simulink model "TransferFunctionAnaylsis"  (R2024a)
settings: Solver=VariableStepAuto  StartTime=0.0  StopTime=10.0  RelTol=1e-3
values from neighbouring files (symbols this model uses):
  Flux = 0.1827    [Parameters.m]    (also in StateSpace.m = 0.192)
  L_d = 0.00525    [Parameters.m]
  L_q = 0.00525    [Parameters.m]
  R_s = 0.9585    [Parameters.m]
libraries: simulink x1
settings Model: Creator=nicco  LastModifiedBy=nicco

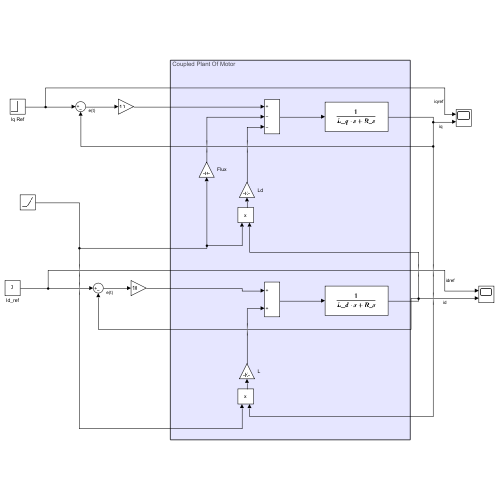
[thumbnail: Simulink's stored preview of the top-level diagram]
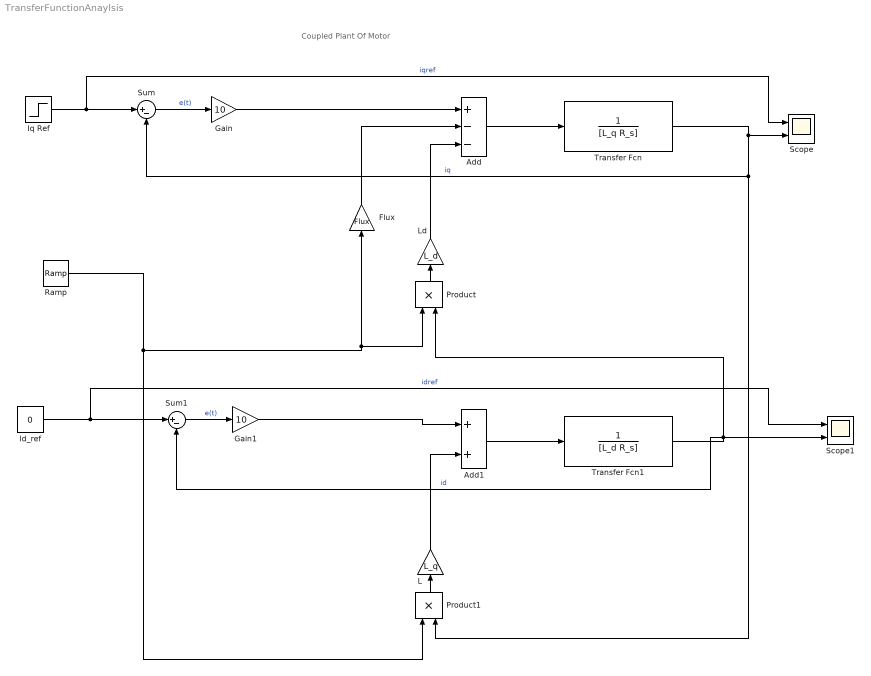
== system TransferFunctionAnaylsis ==
  note: Coupled Plant Of Motor
  Add : Sum  Inputs=+--
  Add1 : Sum
  Flux : Gain  Gain=Flux
  Gain : Gain  Gain=10
  Gain1 : Gain  Gain=10
  Id_ref : Constant  Value=0
  Iq Ref : Step  After=10  SampleTime=0
  L : Gain  Gain=L_q
  Ld : Gain  Gain=L_d
  Product : Product
  Product1 : Product
  Ramp : simulink/Sources/Ramp  slope=10  start=0  InitialOutput=0
  Scope : Scope  NumInputPorts=2
  Scope1 : Scope  NumInputPorts=2
  Sum : Sum  Inputs=|+-
  Sum1 : Sum  Inputs=|+-
  Transfer Fcn : TransferFcn  Denominator=[L_q R_s]
  Transfer Fcn1 : TransferFcn  Denominator=[L_d R_s]
  wires:
  Add/1 -> Transfer Fcn/1
  Flux/1 -> Add/2
  Ld/1 -> Add/3
  Product/1 -> Ld/1
  Transfer Fcn/1 -> Sum/2, Product1/2, Scope/2  "iq"
  Sum/1 -> Gain/1  "e(t)"
  Iq Ref/1 -> Sum/1, Scope/1  "iqref"
  Transfer Fcn1/1 -> Scope1/2, Sum1/2, Product/2  "id"
  Product1/1 -> L/1
  Ramp/1 -> Flux/1, Product/1, Product1/1
  Id_ref/1 -> Sum1/1, Scope1/1  "idref"
  Sum1/1 -> Gain1/1  "e(t)"
  Add1/1 -> Transfer Fcn1/1
  L/1 -> Add1/2
  Gain/1 -> Add/1
  Gain1/1 -> Add1/1
